simulink model "SIFT"  (R2015a)
settings: Solver=ode45  StartTime=0.0  StopTime=10.0  RelTol=1e-3
InitFcn:
  | %% DSPBuilder Start
  | alt_dspbuilder_update_model(bdroot)
  | %% DSPBuilder End
libraries: allblocks_alteradspbuilder2 x2272
(part 24 of 26)

== system SIFT/sift_octave1/matching/compare_descriptor/get_distance5/sub_GradOrian2 ==
  bin1 : Inport
  bin2 : Inport  Port=2
  clken : Inport  Port=3
  Comparator3 : allblocks_alteradspbuilder2/Comparator  direction=a > b  pipeline_display=0  allowFloatingPointOverride=on  logOutputs=off  logFile=C:\Users\ASUS\Desktop\sift_fpga\Octave_2\tb_SIFT\SIFT_sift%5Foctave1_matching_compare%5Fdescriptor_get%5Fdistance5_sub%5FGradOrian2_Comparator3.fixedpointlog
  Delay : allblocks_alteradspbuilder2/Delay  pipeline=1  pipeline_display=1  ClockPhase=1  use_ena=on  use_sclr=off  allowFloatingPointOverride=on  logOutputs=off  logFile=C:\Users\ASUS\Desktop\sift_fpga\Octave_2\tb_SIFT\SIFT_sift%5Foctave1_matching_compare%5Fdescriptor_get%5Fdistance5_sub%5FGradOrian2_Delay.fixedpointlog  use_init=off  reset_value=1
  Multiplexer2 : allblocks_alteradspbuilder2/Multiplexer  numInputs=2  pipeline=0  oneHot=off  pipeline_display=0  use_ena=off  use_aclr=off  allowFloatingPointOverride=on  logOutputs=off  logFile=C:\Users\ASUS\Desktop\sift_fpga\Octave_2\tb_SIFT\SIFT_sift%5Foctave1_matching_compare%5Fdescriptor_get%5Fdistance5_sub%5FGradOrian2_Multiplexer2.fixedpointlog
  Parallel Adder Subtractor : allblocks_alteradspbuilder2/Parallel Adder Subtractor  number_of_inputs=2  direction=+-  use_pipeline=on  pipeline_display=1  phase_selection=1  use_ena=on  use_aclr=off  allowFloatingPointOverride=on  logOutputs=off  logFile=C:\Users\ASUS\Desktop\sift_fpga\Octave_2\tb_SIFT\SIFT_sift%5Foctave1_matching_compare%5Fdescriptor_get%5Fdistance5_sub%5FGradOrian2_Parallel+Adder+Subtractor.fixedpointlog
  Parallel Adder Subtractor1 : allblocks_alteradspbuilder2/Parallel Adder Subtractor  number_of_inputs=2  direction=+-  use_pipeline=on  pipeline_display=1  phase_selection=1  use_ena=on  use_aclr=off  allowFloatingPointOverride=on  logOutputs=off  logFile=C:\Users\ASUS\Desktop\sift_fpga\Octave_2\tb_SIFT\SIFT_sift%5Foctave1_matching_compare%5Fdescriptor_get%5Fdistance5_sub%5FGradOrian2_Parallel+Adder+Subtractor1.fixedpointlog
  sub_bin : Outport
  wires:
  Comparator3/1 -> Delay/1
  [bin2] -> Comparator3/2
  [bin1] -> Comparator3/1
  Delay/1 -> Multiplexer2/1
  [clken] -> Delay/2
  [bin2] -> Parallel Adder Subtractor/2
  [bin1] -> Parallel Adder Subtractor1/2
  [bin2] -> Parallel Adder Subtractor1/1
  [clken] -> Parallel Adder Subtractor/3
  Parallel Adder Subtractor/1 -> [bin12]
  Parallel Adder Subtractor1/1 -> [bin21]
  [clken] -> Parallel Adder Subtractor1/3
  [bin1] -> Parallel Adder Subtractor/1
  bin1/1 -> [bin1]
  bin2/1 -> [bin2]
  [bin12] -> Multiplexer2/3
  [bin21] -> Multiplexer2/2
  Multiplexer2/1 -> sub_bin/1
  clken/1 -> [clken]

== system SIFT/sift_octave1/matching/compare_descriptor/get_distance5/sub_GradOrian3 ==
  bin1 : Inport
  bin2 : Inport  Port=2
  clken : Inport  Port=3
  Comparator3 : allblocks_alteradspbuilder2/Comparator  direction=a > b  pipeline_display=0  allowFloatingPointOverride=on  logOutputs=off  logFile=C:\Users\ASUS\Desktop\sift_fpga\Octave_2\tb_SIFT\SIFT_sift%5Foctave1_matching_compare%5Fdescriptor_get%5Fdistance5_sub%5FGradOrian3_Comparator3.fixedpointlog
  Delay : allblocks_alteradspbuilder2/Delay  pipeline=1  pipeline_display=1  ClockPhase=1  use_ena=on  use_sclr=off  allowFloatingPointOverride=on  logOutputs=off  logFile=C:\Users\ASUS\Desktop\sift_fpga\Octave_2\tb_SIFT\SIFT_sift%5Foctave1_matching_compare%5Fdescriptor_get%5Fdistance5_sub%5FGradOrian3_Delay.fixedpointlog  use_init=off  reset_value=1
  Multiplexer2 : allblocks_alteradspbuilder2/Multiplexer  numInputs=2  pipeline=0  oneHot=off  pipeline_display=0  use_ena=off  use_aclr=off  allowFloatingPointOverride=on  logOutputs=off  logFile=C:\Users\ASUS\Desktop\sift_fpga\Octave_2\tb_SIFT\SIFT_sift%5Foctave1_matching_compare%5Fdescriptor_get%5Fdistance5_sub%5FGradOrian3_Multiplexer2.fixedpointlog
  Parallel Adder Subtractor : allblocks_alteradspbuilder2/Parallel Adder Subtractor  number_of_inputs=2  direction=+-  use_pipeline=on  pipeline_display=1  phase_selection=1  use_ena=on  use_aclr=off  allowFloatingPointOverride=on  logOutputs=off  logFile=C:\Users\ASUS\Desktop\sift_fpga\Octave_2\tb_SIFT\SIFT_sift%5Foctave1_matching_compare%5Fdescriptor_get%5Fdistance5_sub%5FGradOrian3_Parallel+Adder+Subtractor.fixedpointlog
  Parallel Adder Subtractor1 : allblocks_alteradspbuilder2/Parallel Adder Subtractor  number_of_inputs=2  direction=+-  use_pipeline=on  pipeline_display=1  phase_selection=1  use_ena=on  use_aclr=off  allowFloatingPointOverride=on  logOutputs=off  logFile=C:\Users\ASUS\Desktop\sift_fpga\Octave_2\tb_SIFT\SIFT_sift%5Foctave1_matching_compare%5Fdescriptor_get%5Fdistance5_sub%5FGradOrian3_Parallel+Adder+Subtractor1.fixedpointlog
  sub_bin : Outport
  wires:
  Comparator3/1 -> Delay/1
  [bin2] -> Comparator3/2
  [bin1] -> Comparator3/1
  Delay/1 -> Multiplexer2/1
  [clken] -> Delay/2
  [bin2] -> Parallel Adder Subtractor/2
  [bin1] -> Parallel Adder Subtractor1/2
  [bin2] -> Parallel Adder Subtractor1/1
  [clken] -> Parallel Adder Subtractor/3
  Parallel Adder Subtractor/1 -> [bin12]
  Parallel Adder Subtractor1/1 -> [bin21]
  [clken] -> Parallel Adder Subtractor1/3
  [bin1] -> Parallel Adder Subtractor/1
  bin1/1 -> [bin1]
  bin2/1 -> [bin2]
  [bin12] -> Multiplexer2/3
  [bin21] -> Multiplexer2/2
  Multiplexer2/1 -> sub_bin/1
  clken/1 -> [clken]

== system SIFT/sift_octave1/matching/compare_descriptor/get_distance5/sub_GradOrian4 ==
  bin1 : Inport
  bin2 : Inport  Port=2
  clken : Inport  Port=3
  Comparator3 : allblocks_alteradspbuilder2/Comparator  direction=a > b  pipeline_display=0  allowFloatingPointOverride=on  logOutputs=off  logFile=C:\Users\ASUS\Desktop\sift_fpga\Octave_2\tb_SIFT\SIFT_sift%5Foctave1_matching_compare%5Fdescriptor_get%5Fdistance5_sub%5FGradOrian4_Comparator3.fixedpointlog
  Delay : allblocks_alteradspbuilder2/Delay  pipeline=1  pipeline_display=1  ClockPhase=1  use_ena=on  use_sclr=off  allowFloatingPointOverride=on  logOutputs=off  logFile=C:\Users\ASUS\Desktop\sift_fpga\Octave_2\tb_SIFT\SIFT_sift%5Foctave1_matching_compare%5Fdescriptor_get%5Fdistance5_sub%5FGradOrian4_Delay.fixedpointlog  use_init=off  reset_value=1
  Multiplexer2 : allblocks_alteradspbuilder2/Multiplexer  numInputs=2  pipeline=0  oneHot=off  pipeline_display=0  use_ena=off  use_aclr=off  allowFloatingPointOverride=on  logOutputs=off  logFile=C:\Users\ASUS\Desktop\sift_fpga\Octave_2\tb_SIFT\SIFT_sift%5Foctave1_matching_compare%5Fdescriptor_get%5Fdistance5_sub%5FGradOrian4_Multiplexer2.fixedpointlog
  Parallel Adder Subtractor : allblocks_alteradspbuilder2/Parallel Adder Subtractor  number_of_inputs=2  direction=+-  use_pipeline=on  pipeline_display=1  phase_selection=1  use_ena=on  use_aclr=off  allowFloatingPointOverride=on  logOutputs=off  logFile=C:\Users\ASUS\Desktop\sift_fpga\Octave_2\tb_SIFT\SIFT_sift%5Foctave1_matching_compare%5Fdescriptor_get%5Fdistance5_sub%5FGradOrian4_Parallel+Adder+Subtractor.fixedpointlog
  Parallel Adder Subtractor1 : allblocks_alteradspbuilder2/Parallel Adder Subtractor  number_of_inputs=2  direction=+-  use_pipeline=on  pipeline_display=1  phase_selection=1  use_ena=on  use_aclr=off  allowFloatingPointOverride=on  logOutputs=off  logFile=C:\Users\ASUS\Desktop\sift_fpga\Octave_2\tb_SIFT\SIFT_sift%5Foctave1_matching_compare%5Fdescriptor_get%5Fdistance5_sub%5FGradOrian4_Parallel+Adder+Subtractor1.fixedpointlog
  sub_bin : Outport
  wires:
  Comparator3/1 -> Delay/1
  [bin2] -> Comparator3/2
  [bin1] -> Comparator3/1
  Delay/1 -> Multiplexer2/1
  [clken] -> Delay/2
  [bin2] -> Parallel Adder Subtractor/2
  [bin1] -> Parallel Adder Subtractor1/2
  [bin2] -> Parallel Adder Subtractor1/1
  [clken] -> Parallel Adder Subtractor/3
  Parallel Adder Subtractor/1 -> [bin12]
  Parallel Adder Subtractor1/1 -> [bin21]
  [clken] -> Parallel Adder Subtractor1/3
  [bin1] -> Parallel Adder Subtractor/1
  bin1/1 -> [bin1]
  bin2/1 -> [bin2]
  [bin12] -> Multiplexer2/3
  [bin21] -> Multiplexer2/2
  Multiplexer2/1 -> sub_bin/1
  clken/1 -> [clken]

== system SIFT/sift_octave1/matching/compare_descriptor/get_distance5/sub_GradOrian5 ==
  bin1 : Inport
  bin2 : Inport  Port=2
  clken : Inport  Port=3
  Comparator3 : allblocks_alteradspbuilder2/Comparator  direction=a > b  pipeline_display=0  allowFloatingPointOverride=on  logOutputs=off  logFile=C:\Users\ASUS\Desktop\sift_fpga\Octave_2\tb_SIFT\SIFT_sift%5Foctave1_matching_compare%5Fdescriptor_get%5Fdistance5_sub%5FGradOrian5_Comparator3.fixedpointlog
  Delay : allblocks_alteradspbuilder2/Delay  pipeline=1  pipeline_display=1  ClockPhase=1  use_ena=on  use_sclr=off  allowFloatingPointOverride=on  logOutputs=off  logFile=C:\Users\ASUS\Desktop\sift_fpga\Octave_2\tb_SIFT\SIFT_sift%5Foctave1_matching_compare%5Fdescriptor_get%5Fdistance5_sub%5FGradOrian5_Delay.fixedpointlog  use_init=off  reset_value=1
  Multiplexer2 : allblocks_alteradspbuilder2/Multiplexer  numInputs=2  pipeline=0  oneHot=off  pipeline_display=0  use_ena=off  use_aclr=off  allowFloatingPointOverride=on  logOutputs=off  logFile=C:\Users\ASUS\Desktop\sift_fpga\Octave_2\tb_SIFT\SIFT_sift%5Foctave1_matching_compare%5Fdescriptor_get%5Fdistance5_sub%5FGradOrian5_Multiplexer2.fixedpointlog
  Parallel Adder Subtractor : allblocks_alteradspbuilder2/Parallel Adder Subtractor  number_of_inputs=2  direction=+-  use_pipeline=on  pipeline_display=1  phase_selection=1  use_ena=on  use_aclr=off  allowFloatingPointOverride=on  logOutputs=off  logFile=C:\Users\ASUS\Desktop\sift_fpga\Octave_2\tb_SIFT\SIFT_sift%5Foctave1_matching_compare%5Fdescriptor_get%5Fdistance5_sub%5FGradOrian5_Parallel+Adder+Subtractor.fixedpointlog
  Parallel Adder Subtractor1 : allblocks_alteradspbuilder2/Parallel Adder Subtractor  number_of_inputs=2  direction=+-  use_pipeline=on  pipeline_display=1  phase_selection=1  use_ena=on  use_aclr=off  allowFloatingPointOverride=on  logOutputs=off  logFile=C:\Users\ASUS\Desktop\sift_fpga\Octave_2\tb_SIFT\SIFT_sift%5Foctave1_matching_compare%5Fdescriptor_get%5Fdistance5_sub%5FGradOrian5_Parallel+Adder+Subtractor1.fixedpointlog
  sub_bin : Outport
  wires:
  Comparator3/1 -> Delay/1
  [bin2] -> Comparator3/2
  [bin1] -> Comparator3/1
  Delay/1 -> Multiplexer2/1
  [clken] -> Delay/2
  [bin2] -> Parallel Adder Subtractor/2
  [bin1] -> Parallel Adder Subtractor1/2
  [bin2] -> Parallel Adder Subtractor1/1
  [clken] -> Parallel Adder Subtractor/3
  Parallel Adder Subtractor/1 -> [bin12]
  Parallel Adder Subtractor1/1 -> [bin21]
  [clken] -> Parallel Adder Subtractor1/3
  [bin1] -> Parallel Adder Subtractor/1
  bin1/1 -> [bin1]
  bin2/1 -> [bin2]
  [bin12] -> Multiplexer2/3
  [bin21] -> Multiplexer2/2
  Multiplexer2/1 -> sub_bin/1
  clken/1 -> [clken]

== system SIFT/sift_octave1/matching/compare_descriptor/get_distance5/sub_GradOrian6 ==
  bin1 : Inport
  bin2 : Inport  Port=2
  clken : Inport  Port=3
  Comparator3 : allblocks_alteradspbuilder2/Comparator  direction=a > b  pipeline_display=0  allowFloatingPointOverride=on  logOutputs=off  logFile=C:\Users\ASUS\Desktop\sift_fpga\Octave_2\tb_SIFT\SIFT_sift%5Foctave1_matching_compare%5Fdescriptor_get%5Fdistance5_sub%5FGradOrian6_Comparator3.fixedpointlog
  Delay : allblocks_alteradspbuilder2/Delay  pipeline=1  pipeline_display=1  ClockPhase=1  use_ena=on  use_sclr=off  allowFloatingPointOverride=on  logOutputs=off  logFile=C:\Users\ASUS\Desktop\sift_fpga\Octave_2\tb_SIFT\SIFT_sift%5Foctave1_matching_compare%5Fdescriptor_get%5Fdistance5_sub%5FGradOrian6_Delay.fixedpointlog  use_init=off  reset_value=1
  Multiplexer2 : allblocks_alteradspbuilder2/Multiplexer  numInputs=2  pipeline=0  oneHot=off  pipeline_display=0  use_ena=off  use_aclr=off  allowFloatingPointOverride=on  logOutputs=off  logFile=C:\Users\ASUS\Desktop\sift_fpga\Octave_2\tb_SIFT\SIFT_sift%5Foctave1_matching_compare%5Fdescriptor_get%5Fdistance5_sub%5FGradOrian6_Multiplexer2.fixedpointlog
  Parallel Adder Subtractor : allblocks_alteradspbuilder2/Parallel Adder Subtractor  number_of_inputs=2  direction=+-  use_pipeline=on  pipeline_display=1  phase_selection=1  use_ena=on  use_aclr=off  allowFloatingPointOverride=on  logOutputs=off  logFile=C:\Users\ASUS\Desktop\sift_fpga\Octave_2\tb_SIFT\SIFT_sift%5Foctave1_matching_compare%5Fdescriptor_get%5Fdistance5_sub%5FGradOrian6_Parallel+Adder+Subtractor.fixedpointlog
  Parallel Adder Subtractor1 : allblocks_alteradspbuilder2/Parallel Adder Subtractor  number_of_inputs=2  direction=+-  use_pipeline=on  pipeline_display=1  phase_selection=1  use_ena=on  use_aclr=off  allowFloatingPointOverride=on  logOutputs=off  logFile=C:\Users\ASUS\Desktop\sift_fpga\Octave_2\tb_SIFT\SIFT_sift%5Foctave1_matching_compare%5Fdescriptor_get%5Fdistance5_sub%5FGradOrian6_Parallel+Adder+Subtractor1.fixedpointlog
  sub_bin : Outport
  wires:
  Comparator3/1 -> Delay/1
  [bin2] -> Comparator3/2
  [bin1] -> Comparator3/1
  Delay/1 -> Multiplexer2/1
  [clken] -> Delay/2
  [bin2] -> Parallel Adder Subtractor/2
  [bin1] -> Parallel Adder Subtractor1/2
  [bin2] -> Parallel Adder Subtractor1/1
  [clken] -> Parallel Adder Subtractor/3
  Parallel Adder Subtractor/1 -> [bin12]
  Parallel Adder Subtractor1/1 -> [bin21]
  [clken] -> Parallel Adder Subtractor1/3
  [bin1] -> Parallel Adder Subtractor/1
  bin1/1 -> [bin1]
  bin2/1 -> [bin2]
  [bin12] -> Multiplexer2/3
  [bin21] -> Multiplexer2/2
  Multiplexer2/1 -> sub_bin/1
  clken/1 -> [clken]

== system SIFT/sift_octave1/matching/compare_descriptor/get_distance5/sub_GradOrian7 ==
  bin1 : Inport
  bin2 : Inport  Port=2
  clken : Inport  Port=3
  Comparator3 : allblocks_alteradspbuilder2/Comparator  direction=a > b  pipeline_display=0  allowFloatingPointOverride=on  logOutputs=off  logFile=C:\Users\ASUS\Desktop\sift_fpga\Octave_2\tb_SIFT\SIFT_sift%5Foctave1_matching_compare%5Fdescriptor_get%5Fdistance5_sub%5FGradOrian7_Comparator3.fixedpointlog
  Delay : allblocks_alteradspbuilder2/Delay  pipeline=1  pipeline_display=1  ClockPhase=1  use_ena=on  use_sclr=off  allowFloatingPointOverride=on  logOutputs=off  logFile=C:\Users\ASUS\Desktop\sift_fpga\Octave_2\tb_SIFT\SIFT_sift%5Foctave1_matching_compare%5Fdescriptor_get%5Fdistance5_sub%5FGradOrian7_Delay.fixedpointlog  use_init=off  reset_value=1
  Multiplexer2 : allblocks_alteradspbuilder2/Multiplexer  numInputs=2  pipeline=0  oneHot=off  pipeline_display=0  use_ena=off  use_aclr=off  allowFloatingPointOverride=on  logOutputs=off  logFile=C:\Users\ASUS\Desktop\sift_fpga\Octave_2\tb_SIFT\SIFT_sift%5Foctave1_matching_compare%5Fdescriptor_get%5Fdistance5_sub%5FGradOrian7_Multiplexer2.fixedpointlog
  Parallel Adder Subtractor : allblocks_alteradspbuilder2/Parallel Adder Subtractor  number_of_inputs=2  direction=+-  use_pipeline=on  pipeline_display=1  phase_selection=1  use_ena=on  use_aclr=off  allowFloatingPointOverride=on  logOutputs=off  logFile=C:\Users\ASUS\Desktop\sift_fpga\Octave_2\tb_SIFT\SIFT_sift%5Foctave1_matching_compare%5Fdescriptor_get%5Fdistance5_sub%5FGradOrian7_Parallel+Adder+Subtractor.fixedpointlog
  Parallel Adder Subtractor1 : allblocks_alteradspbuilder2/Parallel Adder Subtractor  number_of_inputs=2  direction=+-  use_pipeline=on  pipeline_display=1  phase_selection=1  use_ena=on  use_aclr=off  allowFloatingPointOverride=on  logOutputs=off  logFile=C:\Users\ASUS\Desktop\sift_fpga\Octave_2\tb_SIFT\SIFT_sift%5Foctave1_matching_compare%5Fdescriptor_get%5Fdistance5_sub%5FGradOrian7_Parallel+Adder+Subtractor1.fixedpointlog
  sub_bin : Outport
  wires:
  Comparator3/1 -> Delay/1
  [bin2] -> Comparator3/2
  [bin1] -> Comparator3/1
  Delay/1 -> Multiplexer2/1
  [clken] -> Delay/2
  [bin2] -> Parallel Adder Subtractor/2
  [bin1] -> Parallel Adder Subtractor1/2
  [bin2] -> Parallel Adder Subtractor1/1
  [clken] -> Parallel Adder Subtractor/3
  Parallel Adder Subtractor/1 -> [bin12]
  Parallel Adder Subtractor1/1 -> [bin21]
  [clken] -> Parallel Adder Subtractor1/3
  [bin1] -> Parallel Adder Subtractor/1
  bin1/1 -> [bin1]
  bin2/1 -> [bin2]
  [bin12] -> Multiplexer2/3
  [bin21] -> Multiplexer2/2
  Multiplexer2/1 -> sub_bin/1
  clken/1 -> [clken]

== system SIFT/sift_octave1/matching/compare_descriptor/get_distance6/BusSplitter ==
  data_in : Inport
  AltBus : allblocks_alteradspbuilder2/AltBus  BusType=Unsigned Integer  bwl=112  bwr=0  saturate=off  floatingPointInput=on  floatingPointOutput=on  logOutputs=off  logFile=C:\Users\ASUS\Desktop\sift_fpga\Octave_2\tb_SIFT\SIFT_sift%5Foctave1_matching_compare%5Fdescriptor_get%5Fdistance6_BusSplitter_AltBus.fixedpointlog
  AltBus1 : allblocks_alteradspbuilder2/AltBus  BusType=Unsigned Integer  bwl=96  bwr=0  saturate=off  floatingPointInput=on  floatingPointOutput=on  logOutputs=off  logFile=C:\Users\ASUS\Desktop\sift_fpga\Octave_2\tb_SIFT\SIFT_sift%5Foctave1_matching_compare%5Fdescriptor_get%5Fdistance6_BusSplitter_AltBus1.fixedpointlog
  AltBus10 : allblocks_alteradspbuilder2/AltBus  BusType=Unsigned Integer  bwl=16  bwr=0  saturate=off  floatingPointInput=on  floatingPointOutput=on  logOutputs=off  logFile=C:\Users\ASUS\Desktop\sift_fpga\Octave_2\tb_SIFT\SIFT_sift%5Foctave1_matching_compare%5Fdescriptor_get%5Fdistance6_BusSplitter_AltBus10.fixedpointlog
  AltBus11 : allblocks_alteradspbuilder2/AltBus  BusType=Unsigned Integer  bwl=16  bwr=0  saturate=off  floatingPointInput=on  floatingPointOutput=on  logOutputs=off  logFile=C:\Users\ASUS\Desktop\sift_fpga\Octave_2\tb_SIFT\SIFT_sift%5Foctave1_matching_compare%5Fdescriptor_get%5Fdistance6_BusSplitter_AltBus11.fixedpointlog
  AltBus12 : allblocks_alteradspbuilder2/AltBus  BusType=Unsigned Integer  bwl=16  bwr=0  saturate=off  floatingPointInput=on  floatingPointOutput=on  logOutputs=off  logFile=C:\Users\ASUS\Desktop\sift_fpga\Octave_2\tb_SIFT\SIFT_sift%5Foctave1_matching_compare%5Fdescriptor_get%5Fdistance6_BusSplitter_AltBus12.fixedpointlog
  AltBus13 : allblocks_alteradspbuilder2/AltBus  BusType=Unsigned Integer  bwl=16  bwr=0  saturate=off  floatingPointInput=on  floatingPointOutput=on  logOutputs=off  logFile=C:\Users\ASUS\Desktop\sift_fpga\Octave_2\tb_SIFT\SIFT_sift%5Foctave1_matching_compare%5Fdescriptor_get%5Fdistance6_BusSplitter_AltBus13.fixedpointlog
  AltBus2 : allblocks_alteradspbuilder2/AltBus  BusType=Unsigned Integer  bwl=80  bwr=0  saturate=off  floatingPointInput=on  floatingPointOutput=on  logOutputs=off  logFile=C:\Users\ASUS\Desktop\sift_fpga\Octave_2\tb_SIFT\SIFT_sift%5Foctave1_matching_compare%5Fdescriptor_get%5Fdistance6_BusSplitter_AltBus2.fixedpointlog
  AltBus3 : allblocks_alteradspbuilder2/AltBus  BusType=Unsigned Integer  bwl=64  bwr=0  saturate=off  floatingPointInput=on  floatingPointOutput=on  logOutputs=off  logFile=C:\Users\ASUS\Desktop\sift_fpga\Octave_2\tb_SIFT\SIFT_sift%5Foctave1_matching_compare%5Fdescriptor_get%5Fdistance6_BusSplitter_AltBus3.fixedpointlog
  AltBus4 : allblocks_alteradspbuilder2/AltBus  BusType=Unsigned Integer  bwl=48  bwr=0  saturate=off  floatingPointInput=on  floatingPointOutput=on  logOutputs=off  logFile=C:\Users\ASUS\Desktop\sift_fpga\Octave_2\tb_SIFT\SIFT_sift%5Foctave1_matching_compare%5Fdescriptor_get%5Fdistance6_BusSplitter_AltBus4.fixedpointlog
  AltBus5 : allblocks_alteradspbuilder2/AltBus  BusType=Unsigned Integer  bwl=32  bwr=0  saturate=off  floatingPointInput=on  floatingPointOutput=on  logOutputs=off  logFile=C:\Users\ASUS\Desktop\sift_fpga\Octave_2\tb_SIFT\SIFT_sift%5Foctave1_matching_compare%5Fdescriptor_get%5Fdistance6_BusSplitter_AltBus5.fixedpointlog
  AltBus6 : allblocks_alteradspbuilder2/AltBus  BusType=Unsigned Integer  bwl=16  bwr=0  saturate=off  floatingPointInput=on  floatingPointOutput=on  logOutputs=off  logFile=C:\Users\ASUS\Desktop\sift_fpga\Octave_2\tb_SIFT\SIFT_sift%5Foctave1_matching_compare%5Fdescriptor_get%5Fdistance6_BusSplitter_AltBus6.fixedpointlog
  AltBus7 : allblocks_alteradspbuilder2/AltBus  BusType=Unsigned Integer  bwl=16  bwr=0  saturate=off  floatingPointInput=on  floatingPointOutput=on  logOutputs=off  logFile=C:\Users\ASUS\Desktop\sift_fpga\Octave_2\tb_SIFT\SIFT_sift%5Foctave1_matching_compare%5Fdescriptor_get%5Fdistance6_BusSplitter_AltBus7.fixedpointlog
  AltBus8 : allblocks_alteradspbuilder2/AltBus  BusType=Unsigned Integer  bwl=16  bwr=0  saturate=off  floatingPointInput=on  floatingPointOutput=on  logOutputs=off  logFile=C:\Users\ASUS\Desktop\sift_fpga\Octave_2\tb_SIFT\SIFT_sift%5Foctave1_matching_compare%5Fdescriptor_get%5Fdistance6_BusSplitter_AltBus8.fixedpointlog
  AltBus9 : allblocks_alteradspbuilder2/AltBus  BusType=Unsigned Integer  bwl=16  bwr=0  saturate=off  floatingPointInput=on  floatingPointOutput=on  logOutputs=off  logFile=C:\Users\ASUS\Desktop\sift_fpga\Octave_2\tb_SIFT\SIFT_sift%5Foctave1_matching_compare%5Fdescriptor_get%5Fdistance6_BusSplitter_AltBus9.fixedpointlog
  Logical Bus Operator : allblocks_alteradspbuilder2/Logical Bus Operator  BusType=Unsigned Integer  bwl=128  bwr=0  LogicalOp_text=Shift Right  mask_value_num=-5  shift_amount=112  force_sign_ext=off  pipeline_display=0
  Logical Bus Operator1 : allblocks_alteradspbuilder2/Logical Bus Operator  BusType=Unsigned Integer  bwl=112  bwr=0  LogicalOp_text=Shift Right  mask_value_num=-5  shift_amount=96  force_sign_ext=off  pipeline_display=0
  Logical Bus Operator2 : allblocks_alteradspbuilder2/Logical Bus Operator  BusType=Unsigned Integer  bwl=96  bwr=0  LogicalOp_text=Shift Right  mask_value_num=-5  shift_amount=80  force_sign_ext=off  pipeline_display=0
  Logical Bus Operator3 : allblocks_alteradspbuilder2/Logical Bus Operator  BusType=Unsigned Integer  bwl=80  bwr=0  LogicalOp_text=Shift Right  mask_value_num=-5  shift_amount=64  force_sign_ext=off  pipeline_display=0
  Logical Bus Operator4 : allblocks_alteradspbuilder2/Logical Bus Operator  BusType=Unsigned Integer  bwl=64  bwr=0  LogicalOp_text=Shift Right  mask_value_num=-5  shift_amount=48  force_sign_ext=off  pipeline_display=0
  Logical Bus Operator5 : allblocks_alteradspbuilder2/Logical Bus Operator  BusType=Unsigned Integer  bwl=48  bwr=0  LogicalOp_text=Shift Right  mask_value_num=-5  shift_amount=32  force_sign_ext=off  pipeline_display=0
  Logical Bus Operator6 : allblocks_alteradspbuilder2/Logical Bus Operator  BusType=Unsigned Integer  bwl=32  bwr=0  LogicalOp_text=Shift Right  mask_value_num=-5  shift_amount=16  force_sign_ext=off  pipeline_display=0
  bin1 : Outport
  bin2 : Outport  Port=2
  bin3 : Outport  Port=3
  bin4 : Outport  Port=4
  bin5 : Outport  Port=5
  bin6 : Outport  Port=6
  bin7 : Outport  Port=7
  bin8 : Outport  Port=8
  wires:
  Logical Bus Operator6/1 -> AltBus7/1
  AltBus1/1 -> Logical Bus Operator2/1
  AltBus9/1 -> bin5/1
  AltBus8/1 -> bin6/1
  AltBus7/1 -> bin7/1
  AltBus6/1 -> bin8/1
  AltBus/1 -> Logical Bus Operator1/1
  AltBus10/1 -> bin4/1
  AltBus12/1 -> bin3/1
  AltBus11/1 -> bin1/1
  AltBus3/1 -> Logical Bus Operator4/1
  AltBus2/1 -> Logical Bus Operator3/1
  AltBus4/1 -> Logical Bus Operator5/1
  data_in/1 -> AltBus6/1, AltBus5/1, AltBus4/1, AltBus3/1, AltBus2/1, AltBus1/1, AltBus/1, Logical Bus Operator/1
  AltBus5/1 -> Logical Bus Operator6/1
  Logical Bus Operator1/1 -> AltBus13/1
  Logical Bus Operator2/1 -> AltBus12/1
  Logical Bus Operator/1 -> AltBus11/1
  Logical Bus Operator5/1 -> AltBus8/1
  Logical Bus Operator4/1 -> AltBus9/1
  Logical Bus Operator3/1 -> AltBus10/1
  AltBus13/1 -> bin2/1

== system SIFT/sift_octave1/matching/compare_descriptor/get_distance6/BusSplitter1 ==
  data_in : Inport
  AltBus : allblocks_alteradspbuilder2/AltBus  BusType=Unsigned Integer  bwl=112  bwr=0  saturate=off  floatingPointInput=on  floatingPointOutput=on  logOutputs=off  logFile=C:\Users\ASUS\Desktop\sift_fpga\Octave_2\tb_SIFT\SIFT_sift%5Foctave1_matching_compare%5Fdescriptor_get%5Fdistance6_BusSplitter1_AltBus.fixedpointlog
  AltBus1 : allblocks_alteradspbuilder2/AltBus  BusType=Unsigned Integer  bwl=96  bwr=0  saturate=off  floatingPointInput=on  floatingPointOutput=on  logOutputs=off  logFile=C:\Users\ASUS\Desktop\sift_fpga\Octave_2\tb_SIFT\SIFT_sift%5Foctave1_matching_compare%5Fdescriptor_get%5Fdistance6_BusSplitter1_AltBus1.fixedpointlog
  AltBus10 : allblocks_alteradspbuilder2/AltBus  BusType=Unsigned Integer  bwl=16  bwr=0  saturate=off  floatingPointInput=on  floatingPointOutput=on  logOutputs=off  logFile=C:\Users\ASUS\Desktop\sift_fpga\Octave_2\tb_SIFT\SIFT_sift%5Foctave1_matching_compare%5Fdescriptor_get%5Fdistance6_BusSplitter1_AltBus10.fixedpointlog
  AltBus11 : allblocks_alteradspbuilder2/AltBus  BusType=Unsigned Integer  bwl=16  bwr=0  saturate=off  floatingPointInput=on  floatingPointOutput=on  logOutputs=off  logFile=C:\Users\ASUS\Desktop\sift_fpga\Octave_2\tb_SIFT\SIFT_sift%5Foctave1_matching_compare%5Fdescriptor_get%5Fdistance6_BusSplitter1_AltBus11.fixedpointlog
  AltBus12 : allblocks_alteradspbuilder2/AltBus  BusType=Unsigned Integer  bwl=16  bwr=0  saturate=off  floatingPointInput=on  floatingPointOutput=on  logOutputs=off  logFile=C:\Users\ASUS\Desktop\sift_fpga\Octave_2\tb_SIFT\SIFT_sift%5Foctave1_matching_compare%5Fdescriptor_get%5Fdistance6_BusSplitter1_AltBus12.fixedpointlog
  AltBus13 : allblocks_alteradspbuilder2/AltBus  BusType=Unsigned Integer  bwl=16  bwr=0  saturate=off  floatingPointInput=on  floatingPointOutput=on  logOutputs=off  logFile=C:\Users\ASUS\Desktop\sift_fpga\Octave_2\tb_SIFT\SIFT_sift%5Foctave1_matching_compare%5Fdescriptor_get%5Fdistance6_BusSplitter1_AltBus13.fixedpointlog
  AltBus2 : allblocks_alteradspbuilder2/AltBus  BusType=Unsigned Integer  bwl=80  bwr=0  saturate=off  floatingPointInput=on  floatingPointOutput=on  logOutputs=off  logFile=C:\Users\ASUS\Desktop\sift_fpga\Octave_2\tb_SIFT\SIFT_sift%5Foctave1_matching_compare%5Fdescriptor_get%5Fdistance6_BusSplitter1_AltBus2.fixedpointlog
  AltBus3 : allblocks_alteradspbuilder2/AltBus  BusType=Unsigned Integer  bwl=64  bwr=0  saturate=off  floatingPointInput=on  floatingPointOutput=on  logOutputs=off  logFile=C:\Users\ASUS\Desktop\sift_fpga\Octave_2\tb_SIFT\SIFT_sift%5Foctave1_matching_compare%5Fdescriptor_get%5Fdistance6_BusSplitter1_AltBus3.fixedpointlog
  AltBus4 : allblocks_alteradspbuilder2/AltBus  BusType=Unsigned Integer  bwl=48  bwr=0  saturate=off  floatingPointInput=on  floatingPointOutput=on  logOutputs=off  logFile=C:\Users\ASUS\Desktop\sift_fpga\Octave_2\tb_SIFT\SIFT_sift%5Foctave1_matching_compare%5Fdescriptor_get%5Fdistance6_BusSplitter1_AltBus4.fixedpointlog
  AltBus5 : allblocks_alteradspbuilder2/AltBus  BusType=Unsigned Integer  bwl=32  bwr=0  saturate=off  floatingPointInput=on  floatingPointOutput=on  logOutputs=off  logFile=C:\Users\ASUS\Desktop\sift_fpga\Octave_2\tb_SIFT\SIFT_sift%5Foctave1_matching_compare%5Fdescriptor_get%5Fdistance6_BusSplitter1_AltBus5.fixedpointlog
  AltBus6 : allblocks_alteradspbuilder2/AltBus  BusType=Unsigned Integer  bwl=16  bwr=0  saturate=off  floatingPointInput=on  floatingPointOutput=on  logOutputs=off  logFile=C:\Users\ASUS\Desktop\sift_fpga\Octave_2\tb_SIFT\SIFT_sift%5Foctave1_matching_compare%5Fdescriptor_get%5Fdistance6_BusSplitter1_AltBus6.fixedpointlog
  AltBus7 : allblocks_alteradspbuilder2/AltBus  BusType=Unsigned Integer  bwl=16  bwr=0  saturate=off  floatingPointInput=on  floatingPointOutput=on  logOutputs=off  logFile=C:\Users\ASUS\Desktop\sift_fpga\Octave_2\tb_SIFT\SIFT_sift%5Foctave1_matching_compare%5Fdescriptor_get%5Fdistance6_BusSplitter1_AltBus7.fixedpointlog
  AltBus8 : allblocks_alteradspbuilder2/AltBus  BusType=Unsigned Integer  bwl=16  bwr=0  saturate=off  floatingPointInput=on  floatingPointOutput=on  logOutputs=off  logFile=C:\Users\ASUS\Desktop\sift_fpga\Octave_2\tb_SIFT\SIFT_sift%5Foctave1_matching_compare%5Fdescriptor_get%5Fdistance6_BusSplitter1_AltBus8.fixedpointlog
  AltBus9 : allblocks_alteradspbuilder2/AltBus  BusType=Unsigned Integer  bwl=16  bwr=0  saturate=off  floatingPointInput=on  floatingPointOutput=on  logOutputs=off  logFile=C:\Users\ASUS\Desktop\sift_fpga\Octave_2\tb_SIFT\SIFT_sift%5Foctave1_matching_compare%5Fdescriptor_get%5Fdistance6_BusSplitter1_AltBus9.fixedpointlog
  Logical Bus Operator : allblocks_alteradspbuilder2/Logical Bus Operator  BusType=Unsigned Integer  bwl=128  bwr=0  LogicalOp_text=Shift Right  mask_value_num=-5  shift_amount=112  force_sign_ext=off  pipeline_display=0
  Logical Bus Operator1 : allblocks_alteradspbuilder2/Logical Bus Operator  BusType=Unsigned Integer  bwl=112  bwr=0  LogicalOp_text=Shift Right  mask_value_num=-5  shift_amount=96  force_sign_ext=off  pipeline_display=0
  Logical Bus Operator2 : allblocks_alteradspbuilder2/Logical Bus Operator  BusType=Unsigned Integer  bwl=96  bwr=0  LogicalOp_text=Shift Right  mask_value_num=-5  shift_amount=80  force_sign_ext=off  pipeline_display=0
  Logical Bus Operator3 : allblocks_alteradspbuilder2/Logical Bus Operator  BusType=Unsigned Integer  bwl=80  bwr=0  LogicalOp_text=Shift Right  mask_value_num=-5  shift_amount=64  force_sign_ext=off  pipeline_display=0
  Logical Bus Operator4 : allblocks_alteradspbuilder2/Logical Bus Operator  BusType=Unsigned Integer  bwl=64  bwr=0  LogicalOp_text=Shift Right  mask_value_num=-5  shift_amount=48  force_sign_ext=off  pipeline_display=0
  Logical Bus Operator5 : allblocks_alteradspbuilder2/Logical Bus Operator  BusType=Unsigned Integer  bwl=48  bwr=0  LogicalOp_text=Shift Right  mask_value_num=-5  shift_amount=32  force_sign_ext=off  pipeline_display=0
  Logical Bus Operator6 : allblocks_alteradspbuilder2/Logical Bus Operator  BusType=Unsigned Integer  bwl=32  bwr=0  LogicalOp_text=Shift Right  mask_value_num=-5  shift_amount=16  force_sign_ext=off  pipeline_display=0
  bin1 : Outport
  bin2 : Outport  Port=2
  bin3 : Outport  Port=3
  bin4 : Outport  Port=4
  bin5 : Outport  Port=5
  bin6 : Outport  Port=6
  bin7 : Outport  Port=7
  bin8 : Outport  Port=8
  wires:
  Logical Bus Operator6/1 -> AltBus7/1
  AltBus1/1 -> Logical Bus Operator2/1
  AltBus9/1 -> bin5/1
  AltBus8/1 -> bin6/1
  AltBus7/1 -> bin7/1
  AltBus6/1 -> bin8/1
  AltBus/1 -> Logical Bus Operator1/1
  AltBus10/1 -> bin4/1
  AltBus12/1 -> bin3/1
  AltBus11/1 -> bin1/1
  AltBus3/1 -> Logical Bus Operator4/1
  AltBus2/1 -> Logical Bus Operator3/1
  AltBus4/1 -> Logical Bus Operator5/1
  data_in/1 -> AltBus6/1, AltBus5/1, AltBus4/1, AltBus3/1, AltBus2/1, AltBus1/1, AltBus/1, Logical Bus Operator/1
  AltBus5/1 -> Logical Bus Operator6/1
  Logical Bus Operator1/1 -> AltBus13/1
  Logical Bus Operator2/1 -> AltBus12/1
  Logical Bus Operator/1 -> AltBus11/1
  Logical Bus Operator5/1 -> AltBus8/1
  Logical Bus Operator4/1 -> AltBus9/1
  Logical Bus Operator3/1 -> AltBus10/1
  AltBus13/1 -> bin2/1

== system SIFT/sift_octave1/matching/compare_descriptor/get_distance6/sub_GradOrian ==
  bin1 : Inport
  bin2 : Inport  Port=2
  clken : Inport  Port=3
  Comparator3 : allblocks_alteradspbuilder2/Comparator  direction=a > b  pipeline_display=0  allowFloatingPointOverride=on  logOutputs=off  logFile=C:\Users\ASUS\Desktop\sift_fpga\Octave_2\tb_SIFT\SIFT_sift%5Foctave1_matching_compare%5Fdescriptor_get%5Fdistance6_sub%5FGradOrian_Comparator3.fixedpointlog
  Delay : allblocks_alteradspbuilder2/Delay  pipeline=1  pipeline_display=1  ClockPhase=1  use_ena=on  use_sclr=off  allowFloatingPointOverride=on  logOutputs=off  logFile=C:\Users\ASUS\Desktop\sift_fpga\Octave_2\tb_SIFT\SIFT_sift%5Foctave1_matching_compare%5Fdescriptor_get%5Fdistance6_sub%5FGradOrian_Delay.fixedpointlog  use_init=off  reset_value=1
  Multiplexer2 : allblocks_alteradspbuilder2/Multiplexer  numInputs=2  pipeline=0  oneHot=off  pipeline_display=0  use_ena=off  use_aclr=off  allowFloatingPointOverride=on  logOutputs=off  logFile=C:\Users\ASUS\Desktop\sift_fpga\Octave_2\tb_SIFT\SIFT_sift%5Foctave1_matching_compare%5Fdescriptor_get%5Fdistance6_sub%5FGradOrian_Multiplexer2.fixedpointlog
  Parallel Adder Subtractor : allblocks_alteradspbuilder2/Parallel Adder Subtractor  number_of_inputs=2  direction=+-  use_pipeline=on  pipeline_display=1  phase_selection=1  use_ena=on  use_aclr=off  allowFloatingPointOverride=on  logOutputs=off  logFile=C:\Users\ASUS\Desktop\sift_fpga\Octave_2\tb_SIFT\SIFT_sift%5Foctave1_matching_compare%5Fdescriptor_get%5Fdistance6_sub%5FGradOrian_Parallel+Adder+Subtractor.fixedpointlog
  Parallel Adder Subtractor1 : allblocks_alteradspbuilder2/Parallel Adder Subtractor  number_of_inputs=2  direction=+-  use_pipeline=on  pipeline_display=1  phase_selection=1  use_ena=on  use_aclr=off  allowFloatingPointOverride=on  logOutputs=off  logFile=C:\Users\ASUS\Desktop\sift_fpga\Octave_2\tb_SIFT\SIFT_sift%5Foctave1_matching_compare%5Fdescriptor_get%5Fdistance6_sub%5FGradOrian_Parallel+Adder+Subtractor1.fixedpointlog
  sub_bin : Outport
  wires:
  Comparator3/1 -> Delay/1
  [bin2] -> Comparator3/2
  [bin1] -> Comparator3/1
  Delay/1 -> Multiplexer2/1
  [clken] -> Delay/2
  [bin2] -> Parallel Adder Subtractor/2
  [bin1] -> Parallel Adder Subtractor1/2
  [bin2] -> Parallel Adder Subtractor1/1
  [clken] -> Parallel Adder Subtractor/3
  Parallel Adder Subtractor/1 -> [bin12]
  Parallel Adder Subtractor1/1 -> [bin21]
  [clken] -> Parallel Adder Subtractor1/3
  [bin1] -> Parallel Adder Subtractor/1
  bin1/1 -> [bin1]
  bin2/1 -> [bin2]
  [bin12] -> Multiplexer2/3
  [bin21] -> Multiplexer2/2
  Multiplexer2/1 -> sub_bin/1
  clken/1 -> [clken]

== system SIFT/sift_octave1/matching/compare_descriptor/get_distance6/sub_GradOrian1 ==
  bin1 : Inport
  bin2 : Inport  Port=2
  clken : Inport  Port=3
  Comparator3 : allblocks_alteradspbuilder2/Comparator  direction=a > b  pipeline_display=0  allowFloatingPointOverride=on  logOutputs=off  logFile=C:\Users\ASUS\Desktop\sift_fpga\Octave_2\tb_SIFT\SIFT_sift%5Foctave1_matching_compare%5Fdescriptor_get%5Fdistance6_sub%5FGradOrian1_Comparator3.fixedpointlog
  Delay : allblocks_alteradspbuilder2/Delay  pipeline=1  pipeline_display=1  ClockPhase=1  use_ena=on  use_sclr=off  allowFloatingPointOverride=on  logOutputs=off  logFile=C:\Users\ASUS\Desktop\sift_fpga\Octave_2\tb_SIFT\SIFT_sift%5Foctave1_matching_compare%5Fdescriptor_get%5Fdistance6_sub%5FGradOrian1_Delay.fixedpointlog  use_init=off  reset_value=1
  Multiplexer2 : allblocks_alteradspbuilder2/Multiplexer  numInputs=2  pipeline=0  oneHot=off  pipeline_display=0  use_ena=off  use_aclr=off  allowFloatingPointOverride=on  logOutputs=off  logFile=C:\Users\ASUS\Desktop\sift_fpga\Octave_2\tb_SIFT\SIFT_sift%5Foctave1_matching_compare%5Fdescriptor_get%5Fdistance6_sub%5FGradOrian1_Multiplexer2.fixedpointlog
  Parallel Adder Subtractor : allblocks_alteradspbuilder2/Parallel Adder Subtractor  number_of_inputs=2  direction=+-  use_pipeline=on  pipeline_display=1  phase_selection=1  use_ena=on  use_aclr=off  allowFloatingPointOverride=on  logOutputs=off  logFile=C:\Users\ASUS\Desktop\sift_fpga\Octave_2\tb_SIFT\SIFT_sift%5Foctave1_matching_compare%5Fdescriptor_get%5Fdistance6_sub%5FGradOrian1_Parallel+Adder+Subtractor.fixedpointlog
  Parallel Adder Subtractor1 : allblocks_alteradspbuilder2/Parallel Adder Subtractor  number_of_inputs=2  direction=+-  use_pipeline=on  pipeline_display=1  phase_selection=1  use_ena=on  use_aclr=off  allowFloatingPointOverride=on  logOutputs=off  logFile=C:\Users\ASUS\Desktop\sift_fpga\Octave_2\tb_SIFT\SIFT_sift%5Foctave1_matching_compare%5Fdescriptor_get%5Fdistance6_sub%5FGradOrian1_Parallel+Adder+Subtractor1.fixedpointlog
  sub_bin : Outport
  wires:
  Comparator3/1 -> Delay/1
  [bin2] -> Comparator3/2
  [bin1] -> Comparator3/1
  Delay/1 -> Multiplexer2/1
  [clken] -> Delay/2
  [bin2] -> Parallel Adder Subtractor/2
  [bin1] -> Parallel Adder Subtractor1/2
  [bin2] -> Parallel Adder Subtractor1/1
  [clken] -> Parallel Adder Subtractor/3
  Parallel Adder Subtractor/1 -> [bin12]
  Parallel Adder Subtractor1/1 -> [bin21]
  [clken] -> Parallel Adder Subtractor1/3
  [bin1] -> Parallel Adder Subtractor/1
  bin1/1 -> [bin1]
  bin2/1 -> [bin2]
  [bin12] -> Multiplexer2/3
  [bin21] -> Multiplexer2/2
  Multiplexer2/1 -> sub_bin/1
  clken/1 -> [clken]

== system SIFT/sift_octave1/matching/compare_descriptor/get_distance6/sub_GradOrian2 ==
  bin1 : Inport
  bin2 : Inport  Port=2
  clken : Inport  Port=3
  Comparator3 : allblocks_alteradspbuilder2/Comparator  direction=a > b  pipeline_display=0  allowFloatingPointOverride=on  logOutputs=off  logFile=C:\Users\ASUS\Desktop\sift_fpga\Octave_2\tb_SIFT\SIFT_sift%5Foctave1_matching_compare%5Fdescriptor_get%5Fdistance6_sub%5FGradOrian2_Comparator3.fixedpointlog
  Delay : allblocks_alteradspbuilder2/Delay  pipeline=1  pipeline_display=1  ClockPhase=1  use_ena=on  use_sclr=off  allowFloatingPointOverride=on  logOutputs=off  logFile=C:\Users\ASUS\Desktop\sift_fpga\Octave_2\tb_SIFT\SIFT_sift%5Foctave1_matching_compare%5Fdescriptor_get%5Fdistance6_sub%5FGradOrian2_Delay.fixedpointlog  use_init=off  reset_value=1
  Multiplexer2 : allblocks_alteradspbuilder2/Multiplexer  numInputs=2  pipeline=0  oneHot=off  pipeline_display=0  use_ena=off  use_aclr=off  allowFloatingPointOverride=on  logOutputs=off  logFile=C:\Users\ASUS\Desktop\sift_fpga\Octave_2\tb_SIFT\SIFT_sift%5Foctave1_matching_compare%5Fdescriptor_get%5Fdistance6_sub%5FGradOrian2_Multiplexer2.fixedpointlog
  Parallel Adder Subtractor : allblocks_alteradspbuilder2/Parallel Adder Subtractor  number_of_inputs=2  direction=+-  use_pipeline=on  pipeline_display=1  phase_selection=1  use_ena=on  use_aclr=off  allowFloatingPointOverride=on  logOutputs=off  logFile=C:\Users\ASUS\Desktop\sift_fpga\Octave_2\tb_SIFT\SIFT_sift%5Foctave1_matching_compare%5Fdescriptor_get%5Fdistance6_sub%5FGradOrian2_Parallel+Adder+Subtractor.fixedpointlog
  Parallel Adder Subtractor1 : allblocks_alteradspbuilder2/Parallel Adder Subtractor  number_of_inputs=2  direction=+-  use_pipeline=on  pipeline_display=1  phase_selection=1  use_ena=on  use_aclr=off  allowFloatingPointOverride=on  logOutputs=off  logFile=C:\Users\ASUS\Desktop\sift_fpga\Octave_2\tb_SIFT\SIFT_sift%5Foctave1_matching_compare%5Fdescriptor_get%5Fdistance6_sub%5FGradOrian2_Parallel+Adder+Subtractor1.fixedpointlog
  sub_bin : Outport
  wires:
  Comparator3/1 -> Delay/1
  [bin2] -> Comparator3/2
  [bin1] -> Comparator3/1
  Delay/1 -> Multiplexer2/1
  [clken] -> Delay/2
  [bin2] -> Parallel Adder Subtractor/2
  [bin1] -> Parallel Adder Subtractor1/2
  [bin2] -> Parallel Adder Subtractor1/1
  [clken] -> Parallel Adder Subtractor/3
  Parallel Adder Subtractor/1 -> [bin12]
  Parallel Adder Subtractor1/1 -> [bin21]
  [clken] -> Parallel Adder Subtractor1/3
  [bin1] -> Parallel Adder Subtractor/1
  bin1/1 -> [bin1]
  bin2/1 -> [bin2]
  [bin12] -> Multiplexer2/3
  [bin21] -> Multiplexer2/2
  Multiplexer2/1 -> sub_bin/1
  clken/1 -> [clken]

== system SIFT/sift_octave1/matching/compare_descriptor/get_distance6/sub_GradOrian3 ==
  bin1 : Inport
  bin2 : Inport  Port=2
  clken : Inport  Port=3
  Comparator3 : allblocks_alteradspbuilder2/Comparator  direction=a > b  pipeline_display=0  allowFloatingPointOverride=on  logOutputs=off  logFile=C:\Users\ASUS\Desktop\sift_fpga\Octave_2\tb_SIFT\SIFT_sift%5Foctave1_matching_compare%5Fdescriptor_get%5Fdistance6_sub%5FGradOrian3_Comparator3.fixedpointlog
  Delay : allblocks_alteradspbuilder2/Delay  pipeline=1  pipeline_display=1  ClockPhase=1  use_ena=on  use_sclr=off  allowFloatingPointOverride=on  logOutputs=off  logFile=C:\Users\ASUS\Desktop\sift_fpga\Octave_2\tb_SIFT\SIFT_sift%5Foctave1_matching_compare%5Fdescriptor_get%5Fdistance6_sub%5FGradOrian3_Delay.fixedpointlog  use_init=off  reset_value=1
  Multiplexer2 : allblocks_alteradspbuilder2/Multiplexer  numInputs=2  pipeline=0  oneHot=off  pipeline_display=0  use_ena=off  use_aclr=off  allowFloatingPointOverride=on  logOutputs=off  logFile=C:\Users\ASUS\Desktop\sift_fpga\Octave_2\tb_SIFT\SIFT_sift%5Foctave1_matching_compare%5Fdescriptor_get%5Fdistance6_sub%5FGradOrian3_Multiplexer2.fixedpointlog
  Parallel Adder Subtractor : allblocks_alteradspbuilder2/Parallel Adder Subtractor  number_of_inputs=2  direction=+-  use_pipeline=on  pipeline_display=1  phase_selection=1  use_ena=on  use_aclr=off  allowFloatingPointOverride=on  logOutputs=off  logFile=C:\Users\ASUS\Desktop\sift_fpga\Octave_2\tb_SIFT\SIFT_sift%5Foctave1_matching_compare%5Fdescriptor_get%5Fdistance6_sub%5FGradOrian3_Parallel+Adder+Subtractor.fixedpointlog
  Parallel Adder Subtractor1 : allblocks_alteradspbuilder2/Parallel Adder Subtractor  number_of_inputs=2  direction=+-  use_pipeline=on  pipeline_display=1  phase_selection=1  use_ena=on  use_aclr=off  allowFloatingPointOverride=on  logOutputs=off  logFile=C:\Users\ASUS\Desktop\sift_fpga\Octave_2\tb_SIFT\SIFT_sift%5Foctave1_matching_compare%5Fdescriptor_get%5Fdistance6_sub%5FGradOrian3_Parallel+Adder+Subtractor1.fixedpointlog
  sub_bin : Outport
  wires:
  Comparator3/1 -> Delay/1
  [bin2] -> Comparator3/2
  [bin1] -> Comparator3/1
  Delay/1 -> Multiplexer2/1
  [clken] -> Delay/2
  [bin2] -> Parallel Adder Subtractor/2
  [bin1] -> Parallel Adder Subtractor1/2
  [bin2] -> Parallel Adder Subtractor1/1
  [clken] -> Parallel Adder Subtractor/3
  Parallel Adder Subtractor/1 -> [bin12]
  Parallel Adder Subtractor1/1 -> [bin21]
  [clken] -> Parallel Adder Subtractor1/3
  [bin1] -> Parallel Adder Subtractor/1
  bin1/1 -> [bin1]
  bin2/1 -> [bin2]
  [bin12] -> Multiplexer2/3
  [bin21] -> Multiplexer2/2
  Multiplexer2/1 -> sub_bin/1
  clken/1 -> [clken]

== system SIFT/sift_octave1/matching/compare_descriptor/get_distance6/sub_GradOrian4 ==
  bin1 : Inport
  bin2 : Inport  Port=2
  clken : Inport  Port=3
  Comparator3 : allblocks_alteradspbuilder2/Comparator  direction=a > b  pipeline_display=0  allowFloatingPointOverride=on  logOutputs=off  logFile=C:\Users\ASUS\Desktop\sift_fpga\Octave_2\tb_SIFT\SIFT_sift%5Foctave1_matching_compare%5Fdescriptor_get%5Fdistance6_sub%5FGradOrian4_Comparator3.fixedpointlog
  Delay : allblocks_alteradspbuilder2/Delay  pipeline=1  pipeline_display=1  ClockPhase=1  use_ena=on  use_sclr=off  allowFloatingPointOverride=on  logOutputs=off  logFile=C:\Users\ASUS\Desktop\sift_fpga\Octave_2\tb_SIFT\SIFT_sift%5Foctave1_matching_compare%5Fdescriptor_get%5Fdistance6_sub%5FGradOrian4_Delay.fixedpointlog  use_init=off  reset_value=1
  Multiplexer2 : allblocks_alteradspbuilder2/Multiplexer  numInputs=2  pipeline=0  oneHot=off  pipeline_display=0  use_ena=off  use_aclr=off  allowFloatingPointOverride=on  logOutputs=off  logFile=C:\Users\ASUS\Desktop\sift_fpga\Octave_2\tb_SIFT\SIFT_sift%5Foctave1_matching_compare%5Fdescriptor_get%5Fdistance6_sub%5FGradOrian4_Multiplexer2.fixedpointlog
  Parallel Adder Subtractor : allblocks_alteradspbuilder2/Parallel Adder Subtractor  number_of_inputs=2  direction=+-  use_pipeline=on  pipeline_display=1  phase_selection=1  use_ena=on  use_aclr=off  allowFloatingPointOverride=on  logOutputs=off  logFile=C:\Users\ASUS\Desktop\sift_fpga\Octave_2\tb_SIFT\SIFT_sift%5Foctave1_matching_compare%5Fdescriptor_get%5Fdistance6_sub%5FGradOrian4_Parallel+Adder+Subtractor.fixedpointlog
  Parallel Adder Subtractor1 : allblocks_alteradspbuilder2/Parallel Adder Subtractor  number_of_inputs=2  direction=+-  use_pipeline=on  pipeline_display=1  phase_selection=1  use_ena=on  use_aclr=off  allowFloatingPointOverride=on  logOutputs=off  logFile=C:\Users\ASUS\Desktop\sift_fpga\Octave_2\tb_SIFT\SIFT_sift%5Foctave1_matching_compare%5Fdescriptor_get%5Fdistance6_sub%5FGradOrian4_Parallel+Adder+Subtractor1.fixedpointlog
  sub_bin : Outport
  wires:
  Comparator3/1 -> Delay/1
  [bin2] -> Comparator3/2
  [bin1] -> Comparator3/1
  Delay/1 -> Multiplexer2/1
  [clken] -> Delay/2
  [bin2] -> Parallel Adder Subtractor/2
  [bin1] -> Parallel Adder Subtractor1/2
  [bin2] -> Parallel Adder Subtractor1/1
  [clken] -> Parallel Adder Subtractor/3
  Parallel Adder Subtractor/1 -> [bin12]
  Parallel Adder Subtractor1/1 -> [bin21]
  [clken] -> Parallel Adder Subtractor1/3
  [bin1] -> Parallel Adder Subtractor/1
  bin1/1 -> [bin1]
  bin2/1 -> [bin2]
  [bin12] -> Multiplexer2/3
  [bin21] -> Multiplexer2/2
  Multiplexer2/1 -> sub_bin/1
  clken/1 -> [clken]

== system SIFT/sift_octave1/matching/compare_descriptor/get_distance6/sub_GradOrian5 ==
  bin1 : Inport
  bin2 : Inport  Port=2
  clken : Inport  Port=3
  Comparator3 : allblocks_alteradspbuilder2/Comparator  direction=a > b  pipeline_display=0  allowFloatingPointOverride=on  logOutputs=off  logFile=C:\Users\ASUS\Desktop\sift_fpga\Octave_2\tb_SIFT\SIFT_sift%5Foctave1_matching_compare%5Fdescriptor_get%5Fdistance6_sub%5FGradOrian5_Comparator3.fixedpointlog
  Delay : allblocks_alteradspbuilder2/Delay  pipeline=1  pipeline_display=1  ClockPhase=1  use_ena=on  use_sclr=off  allowFloatingPointOverride=on  logOutputs=off  logFile=C:\Users\ASUS\Desktop\sift_fpga\Octave_2\tb_SIFT\SIFT_sift%5Foctave1_matching_compare%5Fdescriptor_get%5Fdistance6_sub%5FGradOrian5_Delay.fixedpointlog  use_init=off  reset_value=1
  Multiplexer2 : allblocks_alteradspbuilder2/Multiplexer  numInputs=2  pipeline=0  oneHot=off  pipeline_display=0  use_ena=off  use_aclr=off  allowFloatingPointOverride=on  logOutputs=off  logFile=C:\Users\ASUS\Desktop\sift_fpga\Octave_2\tb_SIFT\SIFT_sift%5Foctave1_matching_compare%5Fdescriptor_get%5Fdistance6_sub%5FGradOrian5_Multiplexer2.fixedpointlog
  Parallel Adder Subtractor : allblocks_alteradspbuilder2/Parallel Adder Subtractor  number_of_inputs=2  direction=+-  use_pipeline=on  pipeline_display=1  phase_selection=1  use_ena=on  use_aclr=off  allowFloatingPointOverride=on  logOutputs=off  logFile=C:\Users\ASUS\Desktop\sift_fpga\Octave_2\tb_SIFT\SIFT_sift%5Foctave1_matching_compare%5Fdescriptor_get%5Fdistance6_sub%5FGradOrian5_Parallel+Adder+Subtractor.fixedpointlog
  Parallel Adder Subtractor1 : allblocks_alteradspbuilder2/Parallel Adder Subtractor  number_of_inputs=2  direction=+-  use_pipeline=on  pipeline_display=1  phase_selection=1  use_ena=on  use_aclr=off  allowFloatingPointOverride=on  logOutputs=off  logFile=C:\Users\ASUS\Desktop\sift_fpga\Octave_2\tb_SIFT\SIFT_sift%5Foctave1_matching_compare%5Fdescriptor_get%5Fdistance6_sub%5FGradOrian5_Parallel+Adder+Subtractor1.fixedpointlog
  sub_bin : Outport
  wires:
  Comparator3/1 -> Delay/1
  [bin2] -> Comparator3/2
  [bin1] -> Comparator3/1
  Delay/1 -> Multiplexer2/1
  [clken] -> Delay/2
  [bin2] -> Parallel Adder Subtractor/2
  [bin1] -> Parallel Adder Subtractor1/2
  [bin2] -> Parallel Adder Subtractor1/1
  [clken] -> Parallel Adder Subtractor/3
  Parallel Adder Subtractor/1 -> [bin12]
  Parallel Adder Subtractor1/1 -> [bin21]
  [clken] -> Parallel Adder Subtractor1/3
  [bin1] -> Parallel Adder Subtractor/1
  bin1/1 -> [bin1]
  bin2/1 -> [bin2]
  [bin12] -> Multiplexer2/3
  [bin21] -> Multiplexer2/2
  Multiplexer2/1 -> sub_bin/1
  clken/1 -> [clken]

== system SIFT/sift_octave1/matching/compare_descriptor/get_distance6/sub_GradOrian6 ==
  bin1 : Inport
  bin2 : Inport  Port=2
  clken : Inport  Port=3
  Comparator3 : allblocks_alteradspbuilder2/Comparator  direction=a > b  pipeline_display=0  allowFloatingPointOverride=on  logOutputs=off  logFile=C:\Users\ASUS\Desktop\sift_fpga\Octave_2\tb_SIFT\SIFT_sift%5Foctave1_matching_compare%5Fdescriptor_get%5Fdistance6_sub%5FGradOrian6_Comparator3.fixedpointlog
  Delay : allblocks_alteradspbuilder2/Delay  pipeline=1  pipeline_display=1  ClockPhase=1  use_ena=on  use_sclr=off  allowFloatingPointOverride=on  logOutputs=off  logFile=C:\Users\ASUS\Desktop\sift_fpga\Octave_2\tb_SIFT\SIFT_sift%5Foctave1_matching_compare%5Fdescriptor_get%5Fdistance6_sub%5FGradOrian6_Delay.fixedpointlog  use_init=off  reset_value=1
  Multiplexer2 : allblocks_alteradspbuilder2/Multiplexer  numInputs=2  pipeline=0  oneHot=off  pipeline_display=0  use_ena=off  use_aclr=off  allowFloatingPointOverride=on  logOutputs=off  logFile=C:\Users\ASUS\Desktop\sift_fpga\Octave_2\tb_SIFT\SIFT_sift%5Foctave1_matching_compare%5Fdescriptor_get%5Fdistance6_sub%5FGradOrian6_Multiplexer2.fixedpointlog
  Parallel Adder Subtractor : allblocks_alteradspbuilder2/Parallel Adder Subtractor  number_of_inputs=2  direction=+-  use_pipeline=on  pipeline_display=1  phase_selection=1  use_ena=on  use_aclr=off  allowFloatingPointOverride=on  logOutputs=off  logFile=C:\Users\ASUS\Desktop\sift_fpga\Octave_2\tb_SIFT\SIFT_sift%5Foctave1_matching_compare%5Fdescriptor_get%5Fdistance6_sub%5FGradOrian6_Parallel+Adder+Subtractor.fixedpointlog
  Parallel Adder Subtractor1 : allblocks_alteradspbuilder2/Parallel Adder Subtractor  number_of_inputs=2  direction=+-  use_pipeline=on  pipeline_display=1  phase_selection=1  use_ena=on  use_aclr=off  allowFloatingPointOverride=on  logOutputs=off  logFile=C:\Users\ASUS\Desktop\sift_fpga\Octave_2\tb_SIFT\SIFT_sift%5Foctave1_matching_compare%5Fdescriptor_get%5Fdistance6_sub%5FGradOrian6_Parallel+Adder+Subtractor1.fixedpointlog
  sub_bin : Outport
  wires:
  Comparator3/1 -> Delay/1
  [bin2] -> Comparator3/2
  [bin1] -> Comparator3/1
  Delay/1 -> Multiplexer2/1
  [clken] -> Delay/2
  [bin2] -> Parallel Adder Subtractor/2
  [bin1] -> Parallel Adder Subtractor1/2
  [bin2] -> Parallel Adder Subtractor1/1
  [clken] -> Parallel Adder Subtractor/3
  Parallel Adder Subtractor/1 -> [bin12]
  Parallel Adder Subtractor1/1 -> [bin21]
  [clken] -> Parallel Adder Subtractor1/3
  [bin1] -> Parallel Adder Subtractor/1
  bin1/1 -> [bin1]
  bin2/1 -> [bin2]
  [bin12] -> Multiplexer2/3
  [bin21] -> Multiplexer2/2
  Multiplexer2/1 -> sub_bin/1
  clken/1 -> [clken]
